simulink subsystem "GNC"  (R2025b)
settings: Solver=VariableStepAuto  StartTime=0.0  StopTime=10.0  RelTol=1e-3
model mask{mtqMagneticGain=0, mtqResistance=0, mtqMaxVoltage=0, mtqMaxMagDip=0, mtqAllocationMatrix=0, rwInertia=0, rwMaxTorque=0, rwAllocationMatrix=0, magUpdateFreq=0, refTimePosix=0, omgCelBod=0}
  mask prompts: mtqMagneticGain "Magnetic gain [Am2A-1]"; mtqResistance "Electrical resistance [Ohm]"; mtqMaxVoltage "Maximum voltage [V]"; mtqMaxMagDip "Maximum magnetic dipole [Am-2]"; mtqAllocationMatrix "Allocation matrix"; rwInertia "Inertia moment [kgm2]"; rwMaxTorque "Maximum torque [Nm]"; rwAllocationMatrix "Allocation matrix"; magUpdateFreq "Update frequency [Hz]"; refTimePosix "Reference time for ECI2ECEF conversion (UTC, Posix) [s]"; omgCelBod "Celestial body angular velocity [rads-1]"
settings Model: Creator=antoniohernandez-rodiciomateos  LastModifiedBy=antoniohernandez-rodiciomateos

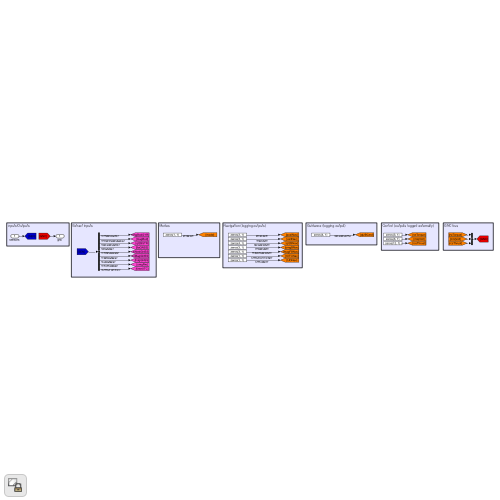
[thumbnail: Simulink's stored preview of the top-level diagram]
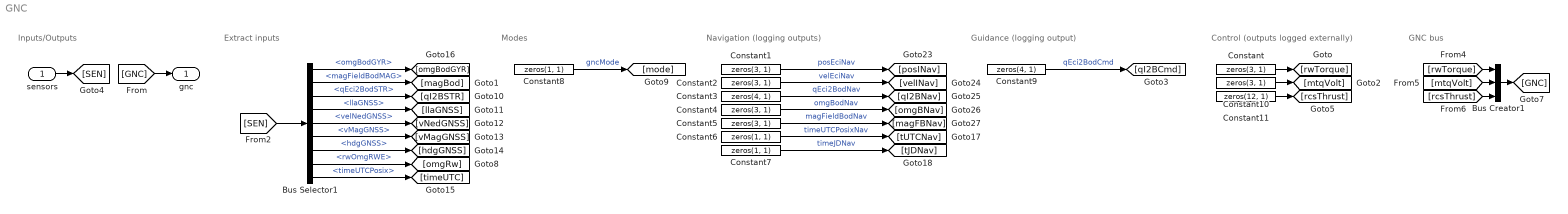
== system GNC ==
  note: Inputs/Outputs
  note: Extract inputs
  note: Modes
  note: Navigation (logging outputs)
  note: Guidance (logging output)
  note: Control (outputs logged externally)
  note: GNC bus
  sensors : Inport  OutDataTypeStr=Bus: sensors_bus
  Bus Creator1 : BusCreator  Inputs=3  OutDataTypeStr=Bus: gnc_bus  NonVirtualBus=on
      settings: InheritFromInputs=off
  Bus Selector1 : BusSelector  OutputSignals=omgBodGYR,magFieldBodMAG,qEci2BodSTR,llaGNSS,velNedGNSS,vMagGNSS,hdgGNSS,rwOmgRWE,timeUTCPosix
  Constant{,1..2,4..5,10} (6 alike) : Constant  Value=zeros(3, 1)
  Constant11 : Constant  Value=zeros(12, 1)
  Constant3 : Constant  Value=zeros(4, 1)
  Constant6 : Constant  Value=zeros(1, 1)
  Constant7 : Constant  Value=zeros(1, 1)
  Constant8 : Constant  Value=zeros(1, 1)
  Constant9 : Constant  Value=zeros(4, 1)
  gnc : Outport  OutDataTypeStr=Bus: gnc_bus
  wires:
  [GNC] -> gnc/1
  sensors/1 -> [SEN]
  [SEN] -> Bus Selector1/1
  Bus Selector1/1 -> [omgBodGYR]  "<omgBodGYR>"
  Bus Selector1/2 -> [magBod]  "<magFieldBodMAG>"
  Bus Selector1/8 -> [omgRw]  "<rwOmgRWE>"
  Bus Selector1/3 -> [qI2BSTR]  "<qEci2BodSTR>"
  Bus Selector1/4 -> [llaGNSS]  "<llaGNSS>"
  Bus Selector1/5 -> [vNedGNSS]  "<velNedGNSS>"
  Bus Selector1/6 -> [vMagGNSS]  "<vMagGNSS>"
  Bus Selector1/7 -> [hdgGNSS]  "<hdgGNSS>"
  Bus Selector1/9 -> [timeUTC]  "<timeUTCPosix>"
  Constant1/1 -> [posINav]  "posEciNav"
  Constant2/1 -> [velINav]  "velEciNav"
  Constant3/1 -> [qI2BNav]  "qEci2BodNav"
  Constant4/1 -> [omgBNav]  "omgBodNav"
  Constant5/1 -> [magFBNav]  "magFieldBodNav"
  Constant6/1 -> [tUTCNav]  "timeUTCPosixNav"
  Constant7/1 -> [tJDNav]  "timeJDNav"
  Constant9/1 -> [qI2BCmd]  "qEci2BodCmd"
  Constant8/1 -> [mode]  "gncMode"
  [rcsThrust] -> Bus Creator1/3
  [mtqVolt] -> Bus Creator1/2
  Bus Creator1/1 -> [GNC]
  [rwTorque] -> Bus Creator1/1
  Constant/1 -> [rwTorque]
  Constant10/1 -> [mtqVolt]
  Constant11/1 -> [rcsThrust]
